simulink model "Final_integration_1"  (R2023b)
settings: Solver=FixedStepAuto  StartTime=0.0  StopTime=inf  FixedStep=Ts  RelTol=1e-3  EnableMultiTasking=on
InitFcn:
  | params
  | pin_params
undefined symbols (not defined in the file or in its folder): b, default1, den_Gd, encoder_scale, f, J, Kb, KD, Kf, KI, Km, KP, L, l, num_Gd, R, r, steering, Vlim
libraries: arduinolib x13, simulink x2, arduinosensorlib x2
settings Model: ExtModeTrigDuration=2  Creator=SJ  LastModifiedBy=SJ
settings SolverCC: AutoInsertRateTranBlk=on
settings OptimizationCC: EnhancedBackFolding=on  PassReuseOutputArgsAs=Individual arguments  ZeroExternalMemoryAtStartup=off  ZeroInternalMemoryAtStartup=off  MaxStackSize=64  OptimizeBlockOrder=speed  DifferentSizesBufferReuse=on  OptimizationCustomize=off  EfficientTunableParamExpr=on
settings DebuggingCC: ParameterTunabilityLossMsg=error
settings HardwareCC: ProdBitPerInt=16  ProdBitPerPointer=16  ProdBitPerSizeT=16  ProdBitPerPtrDiffT=16  ProdLargestAtomicFloat=None  ProdWordSize=8  ProdHWDeviceType=Atmel->AVR
settings SFSimCC: MATLABDynamicMemAlloc=off
settings RTWCC: Description=Embedded Coder  SystemTargetFile=ert.tlc  HardwareBoard=Arduino Mega 2560  TemplateMakefile=ert_default_tmf  Toolchain=Arduino AVR  BuildConfiguration=Faster Runs
settings CodeAppCC: ForceParamTrailComments=on  IgnoreCustomStorageClasses=off  OperatorAnnotations=on  SimulinkDataObjDesc=on  SFDataObjDesc=on  InsertBlockDesc=on
settings ERTTargetCC: SupportContinuousTime=on  SupportVariableSizeSignals=on  ExtModeTransport=3  ExtModeStaticAlloc=on  ExtModeAutomaticAllocSize=off  ExtModeStaticAllocSize=2048  ExtModeMexFile=ext_xcp  ExtModeIntrfLevel=Level2 - Open

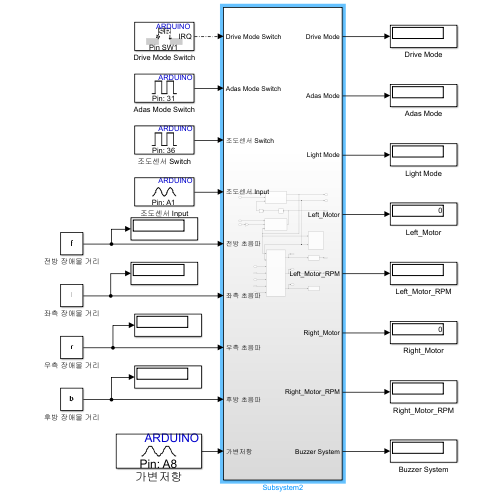
[thumbnail: Simulink's stored preview of the top-level diagram]
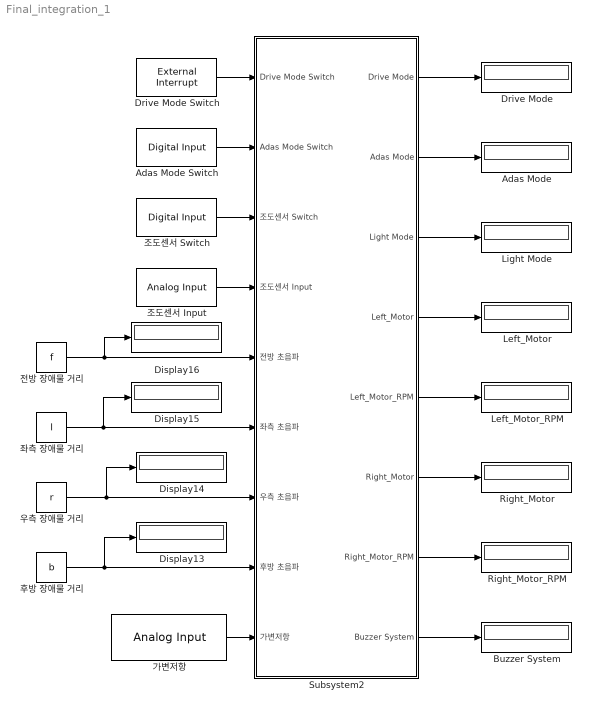
== system Final_integration_1 ==
  Adas Mode : Display
  Adas Mode Switch : arduinolib/Digital Input  pinNumber=SW2  mode=Default  Direction=input  SampleTime=0.01  blockPlatform=arduino
  Buzzer System : Display
  Display{13..16} (4 alike) : Display
  Drive Mode : Display
  Drive Mode Switch : arduinolib/External Interrupt  Pin=SW1  PullUp=off  Mode=RISING  InterruptSimulationInput=off
  Left_Motor : Display
  Left_Motor_RPM : Display
  Light Mode : Display
  Right_Motor : Display
  Right_Motor_RPM : Display
  Subsystem2 : Subsystem
  가변저항 : arduinolib/Analog Input  pinNumber=VR  ReadResultsOnly=off  ConversionTriggerSource=Software  ExternalTriggerType=uint32( 0 )  OutputDataType=uint16  EnableConversionCompleteNotify=off  EnableOuputStatus=off  SampleTime=-1  blockPlatform=arduino
  우측 장애물 거리 : Constant  Value=r
  전방 장애물 거리 : Constant  Value=f
  조도센서 Input : arduinolib/Analog Input  pinNumber=BS  ReadResultsOnly=off  ConversionTriggerSource=Software  ExternalTriggerType=uint32( 0 )  OutputDataType=uint16  EnableConversionCompleteNotify=off  EnableOuputStatus=off  SampleTime=0.01  blockPlatform=arduino
  조도센서 Switch : arduinolib/Digital Input  pinNumber=SW3  mode=Default  Direction=input  SampleTime=0.01  blockPlatform=arduino
  좌측 장애물 거리 : Constant  Value=l
  후방 장애물 거리 : Constant  Value=b
  wires:
  좌측 장애물 거리/1 -> Display15/1, Subsystem2/6(좌측 초음파)
  Subsystem2/7(Right_Motor_RPM) -> Right_Motor_RPM/1
  조도센서 Switch/1 -> Subsystem2/3(조도센서 Switch)
  우측 장애물 거리/1 -> Subsystem2/7(우측 초음파), Display14/1
  가변저항/1 -> Subsystem2/9(가변저항)
  전방 장애물 거리/1 -> Display16/1, Subsystem2/5(전방 초음파)
  조도센서 Input/1 -> Subsystem2/4(조도센서 Input)
  Subsystem2/3(Light Mode) -> Light Mode/1
  Subsystem2/8(Buzzer System) -> Buzzer System/1
  후방 장애물 거리/1 -> Display13/1, Subsystem2/8(후방 초음파)
  Adas Mode Switch/1 -> Subsystem2/2(Adas Mode Switch)
  Subsystem2/4(Left_Motor) -> Left_Motor/1
  Subsystem2/6(Right_Motor) -> Right_Motor/1
  Drive Mode Switch/1 -> Subsystem2/1(Drive Mode Switch)
  Subsystem2/5(Left_Motor_RPM) -> Left_Motor_RPM/1
  Subsystem2/2(Adas Mode) -> Adas Mode/1
  Subsystem2/1(Drive Mode) -> Drive Mode/1

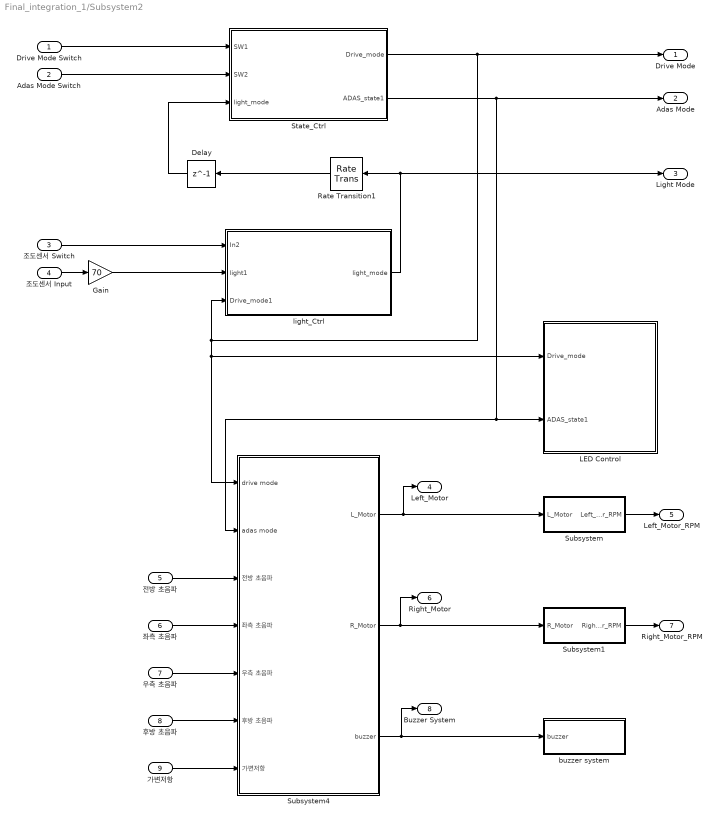
== system Final_integration_1/Subsystem2 ==
  Drive Mode Switch : Inport
  Adas Mode Switch : Inport  Port=2
  조도센서 Switch : Inport  Port=3
  조도센서 Input : Inport  Port=4
  전방 초음파 : Inport  Port=5
  좌측 초음파 : Inport  Port=6
  우측 초음파 : Inport  Port=7
  후방 초음파 : Inport  Port=8
  가변저항 : Inport  Port=9
  Delay : Delay  DelayLength=1
  Gain : Gain  Gain=70
  LED Control : Subsystem
  Rate Transition1 : RateTransition  Integrity=off
  State_Ctrl : Subsystem
  Subsystem : Subsystem
  Subsystem1 : Subsystem
  Subsystem4 : Subsystem
  buzzer system : Subsystem
  light_Ctrl : Subsystem
  Drive Mode : Outport
  Adas Mode : Outport  Port=2
  Light Mode : Outport  Port=3
  Left_Motor : Outport  Port=4
  Left_Motor_RPM : Outport  Port=5
  Right_Motor : Outport  Port=6
  Right_Motor_RPM : Outport  Port=7
  Buzzer System : Outport  Port=8
  wires:
  Subsystem4/1(L_Motor) -> Left_Motor/1, Subsystem/1(L_Motor)
  Subsystem4/3(buzzer) -> Buzzer System/1, buzzer system/1(buzzer)
  light_Ctrl/1(light_mode) -> Rate Transition1/1, Light Mode/1
  Gain/1 -> light_Ctrl/2(light1)
  Rate Transition1/1 -> Delay/1
  Drive Mode Switch/1 -> State_Ctrl/1(SW1)
  Delay/1 -> State_Ctrl/3(light_mode)
  Subsystem4/2(R_Motor) -> Right_Motor/1, Subsystem1/1(R_Motor)
  조도센서 Switch/1 -> light_Ctrl/1(In2)
  Adas Mode Switch/1 -> State_Ctrl/2(SW2)
  조도센서 Input/1 -> Gain/1
  전방 초음파/1 -> Subsystem4/3(전방 초음파)
  가변저항/1 -> Subsystem4/7(가변저항)
  후방 초음파/1 -> Subsystem4/6(후방 초음파)
  좌측 초음파/1 -> Subsystem4/4(좌측 초음파)
  우측 초음파/1 -> Subsystem4/5(우측 초음파)
  Subsystem/1(Left_Motor_RPM) -> Left_Motor_RPM/1
  Subsystem1/1(Right_Motor_RPM) -> Right_Motor_RPM/1
  State_Ctrl/1(Drive_mode) -> Drive Mode/1, Subsystem4/1(drive mode), LED Control/1(Drive_mode), light_Ctrl/3(Drive_mode1)
  State_Ctrl/2(ADAS_state1) -> Subsystem4/2(adas mode), LED Control/2(ADAS_state1), Adas Mode/1

== system Final_integration_1/Subsystem2/LED Control ==
  Drive_mode : Inport
  ADAS_state1 : Inport  Port=2
  LED_B Ctrl : Subsystem
  LED_R Ctrl : Subsystem
  wires:
  ADAS_state1/1 -> LED_B Ctrl/1(ADAS_state)
  Drive_mode/1 -> LED_B Ctrl/2(Drive_mode), LED_R Ctrl/1(Drive_mode)

== system Final_integration_1/Subsystem2/State_Ctrl ==
  SW1 : Inport
  SW2 : Inport  Port=2
  light_mode : Inport  Port=3
  ADAS_state : Subsystem
  Delay : Delay  DelayLength=1
  If : If  IfExpression=u1 ==1  ShowElse=off
  Rate Transition2 : RateTransition  Integrity=off  OutPortSampleTime=0.01
  drive_mode : Subsystem
  Drive_mode : Outport
  ADAS_state1 : Outport  Port=2
  wires:
  If/1 -> ADAS_state/1(In1)
  drive_mode/1(D_mode) -> If/1, Drive_mode/1
  ADAS_state/1(ADAS_state) -> Delay/1, ADAS_state1/1
  SW1/1 -> drive_mode/2(sw1)
  Delay/1 -> drive_mode/3(A_state)
  light_mode/1 -> drive_mode/1(light_mode)
  SW2/1 -> Rate Transition2/1
  Rate Transition2/1 -> ADAS_state/2(In2)

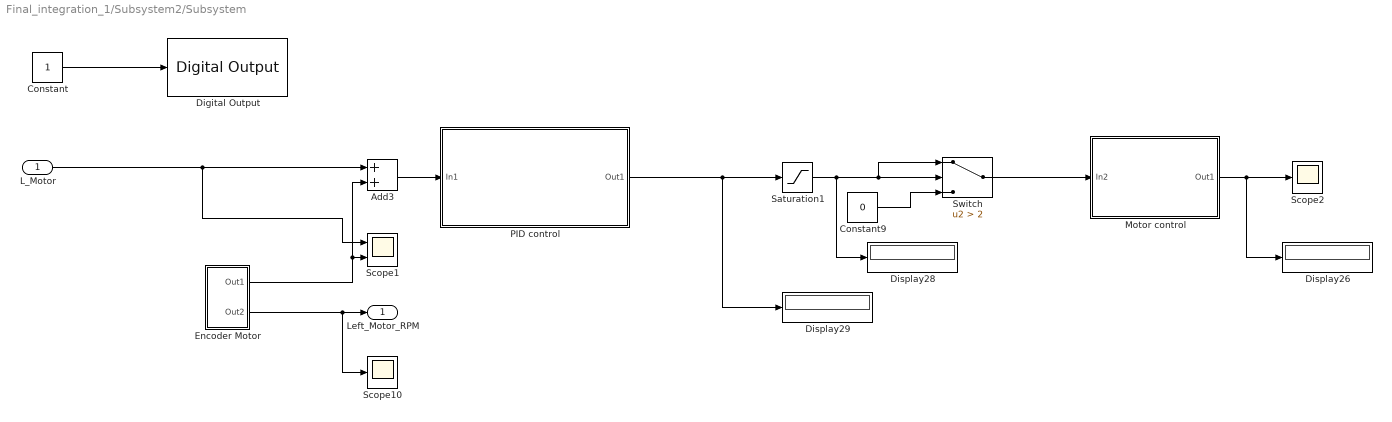
== system Final_integration_1/Subsystem2/Subsystem ==
  L_Motor : Inport
  Add3 : Sum
  Constant : Constant
  Constant9 : Constant  Value=0
  Digital Output : arduinolib/Digital Output  pinNumber=13  Direction=output  blockPlatform=arduino
  Display26 : Display
  Display28 : Display
  Display29 : Display
  Encoder Motor : Subsystem
  Motor control : Subsystem
  PID control : Subsystem
  Saturation1 : Saturate  UpperLimit=12  LowerLimit=2
  Scope1 : Scope  NumInputPorts=2
  Scope10 : Scope
  Scope2 : Scope
  Switch : Switch  Criteria=u2 > Threshold  Threshold=2  SaturateOnIntegerOverflow=off  InputSameDT=off
  Left_Motor_RPM : Outport
  wires:
  L_Motor/1 -> Scope1/1, Add3/1
  Encoder Motor/2(Out2) -> Left_Motor_RPM/1, Scope10/1
  Encoder Motor/1(Out1) -> Add3/2, Scope1/2
  Add3/1 -> PID control/1(In1)
  PID control/1(Out1) -> Display29/1, Saturation1/1
  Saturation1/1 -> Display28/1, Switch/1, Switch/2
  Switch/1 -> Motor control/1(In2)
  Constant9/1 -> Switch/3
  Motor control/1(Out1) -> Scope2/1, Display26/1
  Constant/1 -> Digital Output/1

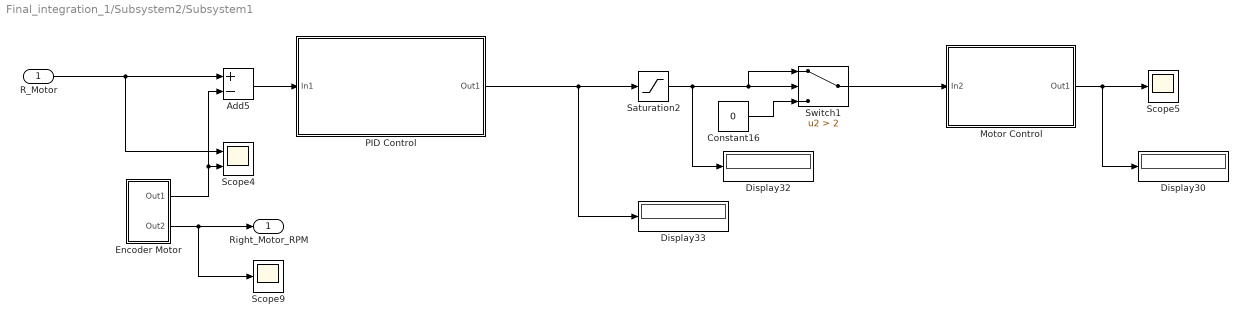
== system Final_integration_1/Subsystem2/Subsystem1 ==
  R_Motor : Inport
  Add5 : Sum  Inputs=+-
  Constant16 : Constant  Value=0
  Display30 : Display
  Display32 : Display
  Display33 : Display
  Encoder Motor : Subsystem
  Motor Control : Subsystem
  PID Control : Subsystem
  Saturation2 : Saturate  UpperLimit=12  LowerLimit=0
  Scope4 : Scope  NumInputPorts=2
  Scope5 : Scope
  Scope9 : Scope
  Switch1 : Switch  Criteria=u2 > Threshold  Threshold=2  SaturateOnIntegerOverflow=off  InputSameDT=off
  Right_Motor_RPM : Outport
  wires:
  Constant16/1 -> Switch1/3
  Switch1/1 -> Motor Control/1(In2)
  Saturation2/1 -> Switch1/1, Switch1/2, Display32/1
  Add5/1 -> PID Control/1(In1)
  R_Motor/1 -> Scope4/1, Add5/1
  Encoder Motor/1(Out1) -> Add5/2, Scope4/2
  PID Control/1(Out1) -> Display33/1, Saturation2/1
  Encoder Motor/2(Out2) -> Right_Motor_RPM/1, Scope9/1
  Motor Control/1(Out1) -> Scope5/1, Display30/1

== system Final_integration_1/Subsystem2/Subsystem4 ==
  drive mode : Inport
  adas mode : Inport  Port=2
  전방 초음파 : Inport  Port=3
  좌측 초음파 : Inport  Port=4
  우측 초음파 : Inport  Port=5
  후방 초음파 : Inport  Port=6
  가변저항 : Inport  Port=7
  Data Type Conversion : DataTypeConversion  OutDataTypeStr=double  SaturateOnIntegerOverflow=off  RndMeth=Floor
  Gain4 : Gain  Gain=0.25
  Subsystem : Subsystem
  L_Motor : Outport
  R_Motor : Outport  Port=2
  buzzer : Outport  Port=3
  wires:
  drive mode/1 -> Subsystem/1(DRIVE MODE1)
  adas mode/1 -> Subsystem/2(ADAS MODE1)
  Subsystem/3(buzzer) -> buzzer/1
  가변저항/1 -> Gain4/1
  Gain4/1 -> Data Type Conversion/1
  Data Type Conversion/1 -> Subsystem/7(가변저항1)
  Subsystem/2(R_Motor1) -> R_Motor/1
  Subsystem/1(L_Motor1) -> L_Motor/1
  전방 초음파/1 -> Subsystem/3(전방 초음파1)
  좌측 초음파/1 -> Subsystem/4(좌측 초음파1)
  우측 초음파/1 -> Subsystem/5(우측 초음파1)
  후방 초음파/1 -> Subsystem/6(후방 초음파1)

== system Final_integration_1/Subsystem2/buzzer system ==
  buzzer : Inport
  If : If  IfExpression=u1 == 1
  If Action Subsystem : Subsystem  TreatAsAtomicUnit=on
  If Action Subsystem1 : Subsystem  TreatAsAtomicUnit=on
  Merge : Merge
  PWM : arduinolib/PWM  pinNumber=Buzzer  frequencyType=Default  desiredFrequency=490.2  achievableFrequency=490.2
  wires:
  buzzer/1 -> If/1
  If/1 -> If Action Subsystem/Action
  If/2 -> If Action Subsystem1/Action
  If Action Subsystem/1(Output) -> Merge/1
  If Action Subsystem1/1(Out1) -> Merge/2
  Merge/1 -> PWM/1

== system Final_integration_1/Subsystem2/light_Ctrl ==
  In2 : Inport
  light1 : Inport  Port=2
  Drive_mode1 : Inport  Port=3
  If : If  IfExpression=u1 == 0  ShowElse=off
  If Action Subsystem : Subsystem  TreatAsAtomicUnit=on
  Rate Transition : RateTransition  Integrity=off
  Rate Transition1 : RateTransition  Integrity=off  OutPortSampleTime=0.2
  Subsystem : Subsystem
  light_mode : Outport
  wires:
  If Action Subsystem/1(light_mode) -> Rate Transition/1
  In2/1 -> Rate Transition1/1
  Rate Transition/1 -> Subsystem/2(light)
  Drive_mode1/1 -> If Action Subsystem/1(Drive_mode1)
  light1/1 -> Subsystem/1(light1)
  Subsystem/1(light_mode) -> light_mode/1
  If/1 -> If Action Subsystem/Action
  Rate Transition1/1 -> If/1

== system Final_integration_1/Subsystem2/LED Control/LED_B Ctrl ==
  ADAS_state : Inport
  Drive_mode : Inport  Port=2
  Constant : Constant
  Digital Output : arduinolib/Digital Output  pinNumber=LED1_B  Direction=output  blockPlatform=arduino
  If Action Subsystem1 : Subsystem  TreatAsAtomicUnit=on
  If Action Subsystem3 : Subsystem  TreatAsAtomicUnit=on
  If1 : If  IfExpression=u1 ==1
  Merge : Merge
  Product : Product
  Product1 : Product
  Pulse Generator : DiscretePulseGenerator  PulseType=Time based  PulseWidth=50
  wires:
  If1/2 -> If Action Subsystem3/Action
  If Action Subsystem1/1(Out1) -> Merge/1
  ADAS_state/1 -> If1/1
  If1/1 -> If Action Subsystem1/Action
  Merge/1 -> Digital Output/1
  If Action Subsystem3/1(Out1) -> Merge/2
  Drive_mode/1 -> Product/1, Product1/2
  Pulse Generator/1 -> Product/2
  Constant/1 -> Product1/1
  Product1/1 -> If Action Subsystem1/1(Input)
  Product/1 -> If Action Subsystem3/1(Input)

== system Final_integration_1/Subsystem2/LED Control/LED_R Ctrl ==
  Drive_mode : Inport
  Digital Output : arduinolib/Digital Output  pinNumber=LED1_R  Direction=output  blockPlatform=arduino
  If Action Subsystem1 : Subsystem  TreatAsAtomicUnit=on
  If Action Subsystem3 : Subsystem  TreatAsAtomicUnit=on
  If1 : If  IfExpression=u1 ==1
  Merge : Merge
  wires:
  If1/2 -> If Action Subsystem3/Action
  If Action Subsystem1/1(Out1) -> Merge/1
  Drive_mode/1 -> If1/1
  If1/1 -> If Action Subsystem1/Action
  Merge/1 -> Digital Output/1
  If Action Subsystem3/1(Out1) -> Merge/2

== system Final_integration_1/Subsystem2/State_Ctrl/ADAS_state ==
  In1 : Inport
  In2 : Inport  Port=2
  If : If  IfExpression=u1 == 0  ShowElse=off
  If Action Subsystem : Subsystem  TreatAsAtomicUnit=on
  If Action Subsystem1 : Subsystem  TreatAsAtomicUnit=on
  Rate Transition : RateTransition  Integrity=off
  Rate Transition2 : RateTransition  Integrity=off  OutPortSampleTime=0.2
  ADAS_state : Outport
  wires:
  In1/1 -> If Action Subsystem/Action
  If Action Subsystem/1(ADAS_state) -> ADAS_state/1
  In2/1 -> Rate Transition2/1
  Rate Transition2/1 -> If/1
  If/1 -> If Action Subsystem1/Action
  If Action Subsystem1/1(sw2) -> Rate Transition/1
  Rate Transition/1 -> If Action Subsystem/1(sw2)

== system Final_integration_1/Subsystem2/State_Ctrl/drive_mode ==
  light_mode : Inport
  sw1 : Inport  Port=2
  A_state : Inport  Port=3
  Rate Transition : RateTransition  Integrity=off  OutPortSampleTime=0.01
  Rate Transition1 : RateTransition  Integrity=off
  Rate Transition2 : RateTransition  Integrity=off
  SW1 : Subsystem
  D_mode : Outport
  wires:
  SW1/1(Output) -> Rate Transition/1
  sw1/1 -> SW1/Trigger
  Rate Transition/1 -> D_mode/1
  light_mode/1 -> Rate Transition1/1
  A_state/1 -> Rate Transition2/1
  Rate Transition1/1 -> SW1/1(light_mode)
  Rate Transition2/1 -> SW1/2(A_state)

== system Final_integration_1/Subsystem2/Subsystem/Encoder Motor ==
  Data Type Conversion1 : DataTypeConversion  OutDataTypeStr=int32  SaturateOnIntegerOverflow=off  RndMeth=Floor
  Discrete Transfer Fcn : DiscreteTransferFcn  Numerator=num_Gd  Denominator=den_Gd
  Discrete Derivative : simulink/Discrete/Discrete Derivative  gainval=1.0  ICPrevScaledInput=0.0  OutMin=[]  OutMax=[]  OutDataType=fixdt(1, 16)  OutScaling=2^-10  DoSatur=off
  Display : Display
  Encoder : arduinosensorlib/Encoder  InputA=L_Encoder_A  InputB=L_Encoder_B  Mode=No reset  SampleTime=0.01
  Gain1 : Gain  Gain=encoder_scale
  Gain2 : Gain  Gain=60/(2*pi)
  Out1 : Outport
  Out2 : Outport  Port=2
  wires:
  Gain1/1 -> Display/1, Gain2/1, Data Type Conversion1/1
  Encoder/1 -> Discrete Derivative/1
  Gain2/1 -> Out2/1
  Data Type Conversion1/1 -> Discrete Transfer Fcn/1
  Discrete Derivative/1 -> Gain1/1
  Discrete Transfer Fcn/1 -> Out1/1

== system Final_integration_1/Subsystem2/Subsystem/Motor control ==
  In2 : Inport
  Add : Sum  Commented=on  Inputs=+-
  Add1 : Sum  Commented=on
  Data Type Conversion : DataTypeConversion  OutDataTypeStr=uint8  SaturateOnIntegerOverflow=off  RndMeth=Floor
  Data Type Conversion1 : DataTypeConversion  OutDataTypeStr=double  SaturateOnIntegerOverflow=off  RndMeth=Floor
  Display1 : Display
  Gain : Gain  Commented=on  Gain=Kb
  Gain1 : Gain  Gain=255/Vlim
  PWM : arduinolib/PWM  pinNumber=Motor_L_Control  frequencyType=Default  desiredFrequency=490.2  achievableFrequency=490.2
  Transfer Fcn : TransferFcn  Commented=on  Numerator=Km  Denominator=[L R]
  Transfer Fcn1 : TransferFcn  Commented=on  Numerator=1  Denominator=[J Kf]
  Out1 : Outport
  wires:
  Add/1 -> Transfer Fcn/1
  Add1/1 -> Transfer Fcn1/1
  Transfer Fcn/1 -> Add1/2
  Gain/1 -> Add/2
  Transfer Fcn1/1 -> Gain/1
  In2/1 -> Gain1/1
  Gain1/1 -> Data Type Conversion/1
  Data Type Conversion1/1 -> Out1/1
  Data Type Conversion/1 -> Data Type Conversion1/1, Display1/1, PWM/1

== system Final_integration_1/Subsystem2/Subsystem/PID control ==
  In1 : Inport
  Add4 : Sum
  Derivative2 : Derivative  Commented=on
  Gain1 : Gain  Commented=on  Gain=KI
  Gain2 : Gain  Commented=on  Gain=KP
  Gain3 : Gain  Commented=on  Gain=KD
  Gain4 : Gain  Gain=KP
  Integrator2 : Integrator  Commented=on
  Subtract2 : Sum  Commented=on  Inputs=+++
  Transfer Fcn1 : TransferFcn  Numerator=[KI]  Denominator=[1 0]
  Out1 : Outport
  wires:
  Add4/1 -> Out1/1
  Gain4/1 -> Add4/2
  Transfer Fcn1/1 -> Add4/1
  Derivative2/1 -> Subtract2/3
  ? -> Gain2/1, Gain3/1, Gain1/1
  Integrator2/1 -> Subtract2/1
  Gain2/1 -> Subtract2/2
  Gain3/1 -> Derivative2/1
  Gain1/1 -> Integrator2/1
  In1/1 -> Gain4/1, Transfer Fcn1/1

== system Final_integration_1/Subsystem2/Subsystem1/Encoder Motor ==
  Data Type Conversion1 : DataTypeConversion  OutDataTypeStr=int32  SaturateOnIntegerOverflow=off  RndMeth=Floor
  Discrete Transfer Fcn : DiscreteTransferFcn  Numerator=num_Gd  Denominator=den_Gd
  Discrete Derivative : simulink/Discrete/Discrete Derivative  gainval=1.0  ICPrevScaledInput=0.0  OutMin=[]  OutMax=[]  OutDataType=fixdt(1, 16)  OutScaling=2^-10  DoSatur=off
  Display : Display
  Encoder : arduinosensorlib/Encoder  InputA=R_Encoder_A  InputB=R_Encoder_B  Mode=No reset  SampleTime=0.01
  Gain1 : Gain  Gain=encoder_scale
  Gain2 : Gain  Gain=60/(2*pi)
  Out1 : Outport
  Out2 : Outport  Port=2
  wires:
  Gain1/1 -> Display/1, Gain2/1, Data Type Conversion1/1
  Encoder/1 -> Discrete Derivative/1
  Gain2/1 -> Out2/1
  Data Type Conversion1/1 -> Discrete Transfer Fcn/1
  Discrete Derivative/1 -> Gain1/1
  Discrete Transfer Fcn/1 -> Out1/1

== system Final_integration_1/Subsystem2/Subsystem1/Motor Control ==
  In2 : Inport
  Add : Sum  Commented=on  Inputs=+-
  Add1 : Sum  Commented=on
  Data Type Conversion : DataTypeConversion  OutDataTypeStr=uint8  SaturateOnIntegerOverflow=off  RndMeth=Floor
  Data Type Conversion1 : DataTypeConversion  OutDataTypeStr=double  SaturateOnIntegerOverflow=off  RndMeth=Floor
  Display1 : Display
  Gain : Gain  Commented=on  Gain=Kb
  Gain1 : Gain  Gain=255/Vlim
  PWM : arduinolib/PWM  pinNumber=Motor_R_control  frequencyType=Default  desiredFrequency=490.2  achievableFrequency=490.2
  Transfer Fcn : TransferFcn  Commented=on  Numerator=Km  Denominator=[L R]
  Transfer Fcn1 : TransferFcn  Commented=on  Numerator=1  Denominator=[J Kf]
  Out1 : Outport
  wires:
  Add/1 -> Transfer Fcn/1
  Add1/1 -> Transfer Fcn1/1
  Transfer Fcn/1 -> Add1/2
  Gain/1 -> Add/2
  Transfer Fcn1/1 -> Gain/1
  In2/1 -> Gain1/1
  Gain1/1 -> Data Type Conversion/1
  Data Type Conversion1/1 -> Out1/1
  Data Type Conversion/1 -> Data Type Conversion1/1, Display1/1, PWM/1

== system Final_integration_1/Subsystem2/Subsystem1/PID Control ==
  In1 : Inport
  Add4 : Sum
  Derivative2 : Derivative  Commented=on
  Gain1 : Gain  Commented=on  Gain=KI
  Gain2 : Gain  Commented=on  Gain=KP
  Gain3 : Gain  Commented=on  Gain=KD
  Gain4 : Gain  Gain=KP
  Integrator2 : Integrator  Commented=on
  Subtract2 : Sum  Commented=on  Inputs=+++
  Transfer Fcn1 : TransferFcn  Numerator=[KI]  Denominator=[1 0]
  Out1 : Outport
  wires:
  Add4/1 -> Out1/1
  Derivative2/1 -> Subtract2/3
  Gain3/1 -> Derivative2/1
  ? -> Gain2/1, Gain3/1, Gain1/1
  Gain2/1 -> Subtract2/2
  Gain1/1 -> Integrator2/1
  Integrator2/1 -> Subtract2/1
  Transfer Fcn1/1 -> Add4/1
  Gain4/1 -> Add4/2
  In1/1 -> Transfer Fcn1/1, Gain4/1

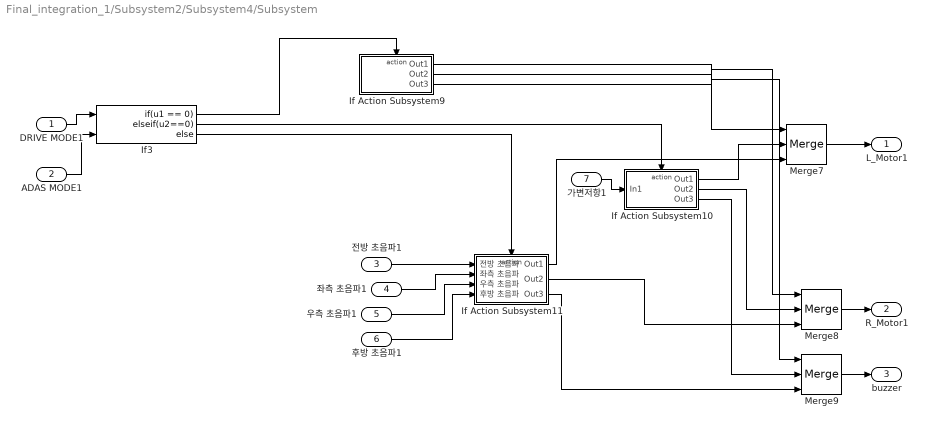
== system Final_integration_1/Subsystem2/Subsystem4/Subsystem ==
  DRIVE MODE1 : Inport
  ADAS MODE1 : Inport  Port=2
  전방 초음파1 : Inport  Port=3
  좌측 초음파1 : Inport  Port=4
  우측 초음파1 : Inport  Port=5
  후방 초음파1 : Inport  Port=6
  가변저항1 : Inport  Port=7
  If Action Subsystem10 : Subsystem  TreatAsAtomicUnit=on
  If Action Subsystem11 : Subsystem  TreatAsAtomicUnit=on
  If Action Subsystem9 : Subsystem  TreatAsAtomicUnit=on
  If3 : If  NumInputs=2  IfExpression=u1 == 0  ElseIfExpressions=u2==0
  Merge7 : Merge  Inputs=3
  Merge8 : Merge  Inputs=3
  Merge9 : Merge  Inputs=3
  L_Motor1 : Outport
  R_Motor1 : Outport  Port=2
  buzzer : Outport  Port=3
  wires:
  후방 초음파1/1 -> If Action Subsystem11/4(후방 초음파)
  Merge9/1 -> buzzer/1
  우측 초음파1/1 -> If Action Subsystem11/3(우측 초음파)
  If Action Subsystem11/1(Out1) -> Merge7/3
  Merge8/1 -> R_Motor1/1
  If Action Subsystem9/2(Out2) -> Merge8/1
  If3/3 -> If Action Subsystem11/Action
  If Action Subsystem10/1(Out1) -> Merge7/2
  Merge7/1 -> L_Motor1/1
  If3/1 -> If Action Subsystem9/Action
  If Action Subsystem9/1(Out1) -> Merge7/1
  If Action Subsystem9/3(Out3) -> Merge9/1
  좌측 초음파1/1 -> If Action Subsystem11/2(좌측 초음파)
  If Action Subsystem11/3(Out3) -> Merge9/3
  전방 초음파1/1 -> If Action Subsystem11/1(전방 초음파)
  If Action Subsystem10/2(Out2) -> Merge8/2
  If Action Subsystem10/3(Out3) -> Merge9/2
  If3/2 -> If Action Subsystem10/Action
  If Action Subsystem11/2(Out2) -> Merge8/3
  DRIVE MODE1/1 -> If3/1
  가변저항1/1 -> If Action Subsystem10/1(In1)
  ADAS MODE1/1 -> If3/2

== system Final_integration_1/Subsystem2/buzzer system/If Action Subsystem ==
  Action Port : ActionPort  ActionPortLabel=if(u1 == 1)
  Pulse Generator : DiscretePulseGenerator  PulseType=Time based  Period=0.2  PulseWidth=50
  Output : Outport
  wires:
  Pulse Generator/1 -> Output/1

== system Final_integration_1/Subsystem2/buzzer system/If Action Subsystem1 ==
  Action Port : ActionPort  ActionPortLabel=else
  Constant : Constant  Value=0
  Out1 : Outport
  wires:
  Constant/1 -> Out1/1

== system Final_integration_1/Subsystem2/light_Ctrl/If Action Subsystem ==
  Drive_mode1 : Inport
  Action Port : ActionPort  ActionPortLabel=if(u1 == 0)
  Constant : Constant
  Constant1 : Constant  Value=3
  Constant2 : Constant  Value=0
  Delay : Delay  DelayLength=1
  If : If  IfExpression=u1 == 1
  If Action Subsystem : Subsystem  TreatAsAtomicUnit=on
  If Action Subsystem1 : Subsystem  TreatAsAtomicUnit=on
  Merge : Merge
  Mod : Math  Operator=mod
  Plus : Sum
  light_mode : Outport
  wires:
  Mod/1 -> light_mode/1, Delay/1
  Delay/1 -> Plus/2
  Plus/1 -> Mod/1
  Constant1/1 -> Mod/2
  If/1 -> If Action Subsystem/Action
  If/2 -> If Action Subsystem1/Action
  Constant/1 -> If Action Subsystem/1(In1)
  Constant2/1 -> If Action Subsystem1/1(In1)
  If Action Subsystem/1(Out1) -> Merge/1
  If Action Subsystem1/1(Out1) -> Merge/2
  Merge/1 -> Plus/1
  Drive_mode1/1 -> If/1

== system Final_integration_1/Subsystem2/light_Ctrl/Subsystem ==
  light1 : Inport
  light : Inport  Port=2
  Chart1 : Stateflow chart  Commented=on  TreatAsAtomicUnit=on
  Subsystem : Subsystem
  light_mode : Outport
  wires:
  light1/1 -> Subsystem/1(light)
  light/1 -> light_mode/1, Subsystem/2(light_mode)

== system Final_integration_1/Subsystem2/LED Control/LED_B Ctrl/If Action Subsystem1 ==
  Input : Inport
  Action Port : ActionPort  ActionPortLabel=if(u1 ==1)
  Out1 : Outport
  wires:
  Input/1 -> Out1/1

== system Final_integration_1/Subsystem2/LED Control/LED_B Ctrl/If Action Subsystem3 ==
  Input : Inport
  Action Port : ActionPort  ActionPortLabel=else
  Out1 : Outport
  wires:
  Input/1 -> Out1/1

== system Final_integration_1/Subsystem2/LED Control/LED_R Ctrl/If Action Subsystem1 ==
  Action Port : ActionPort  ActionPortLabel=if(u1 ==1)
  Constant : Constant
  Out1 : Outport
  wires:
  Constant/1 -> Out1/1

== system Final_integration_1/Subsystem2/LED Control/LED_R Ctrl/If Action Subsystem3 ==
  Action Port : ActionPort  ActionPortLabel=else
  Constant : Constant  Value=0
  Out1 : Outport
  wires:
  Constant/1 -> Out1/1

== system Final_integration_1/Subsystem2/State_Ctrl/ADAS_state/If Action Subsystem ==
  sw2 : Inport
  Action Port : ActionPort  ActionPortLabel=if(u1 ==1)
  ADAS_state : Outport
  wires:
  sw2/1 -> ADAS_state/1

== system Final_integration_1/Subsystem2/State_Ctrl/ADAS_state/If Action Subsystem1 ==
  Action Port : ActionPort  ActionPortLabel=if(u1 == 0)
  Constant2 : Constant
  Constant3 : Constant  Value=2
  Delay1 : Delay  DelayLength=1  InitialCondition=0
  Mod1 : Math  Operator=mod
  Sum : Sum  Inputs=|++
  sw2 : Outport
  wires:
  Mod1/1 -> sw2/1
  Delay1/1 -> Sum/2
  Constant3/1 -> Mod1/2
  Sum/1 -> Delay1/1, Mod1/1
  Constant2/1 -> Sum/1

== system Final_integration_1/Subsystem2/State_Ctrl/drive_mode/SW1 ==
  light_mode : Inport
  A_state : Inport  Port=2
  function : TriggerPort  TriggerType=function-call  VariantControl=(inherit)
  Constant2 : Constant
  Delay : Delay  DelayLength=1
  If : If  IfExpression=u1 == 0  ElseIfExpressions=u1 == 1  ShowElse=off
  If Action Subsystem : Subsystem  TreatAsAtomicUnit=on
  If Action Subsystem1 : Subsystem  TreatAsAtomicUnit=on
  Merge : Merge
  Output : Outport
  wires:
  Delay/1 -> If/1
  If/1 -> If Action Subsystem/Action
  Constant2/1 -> If Action Subsystem/1(In1)
  If/2 -> If Action Subsystem1/Action
  If Action Subsystem/1(Out1) -> Merge/1
  light_mode/1 -> If Action Subsystem1/1(light_mode)
  A_state/1 -> If Action Subsystem1/2(A_state)
  If Action Subsystem1/1(Out1) -> Merge/2
  Merge/1 -> Delay/1, Output/1

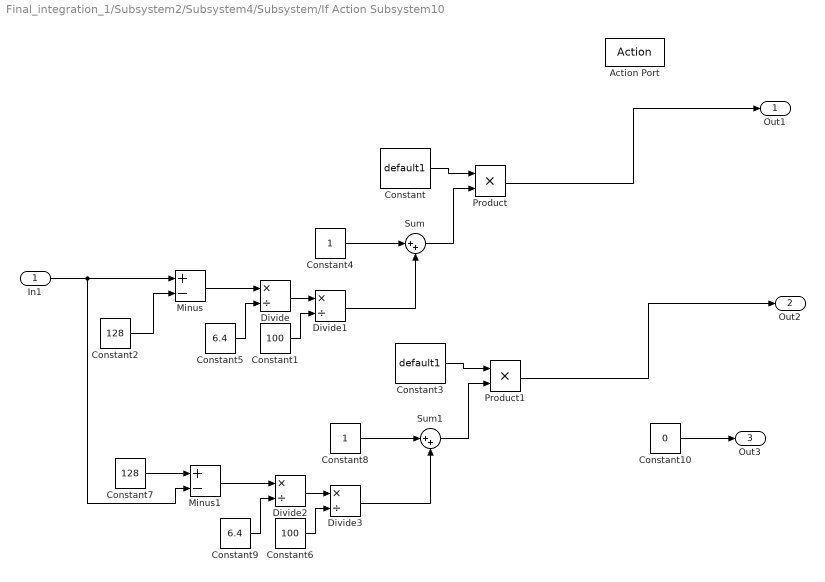
== system Final_integration_1/Subsystem2/Subsystem4/Subsystem/If Action Subsystem10 ==
  In1 : Inport
  Action Port : ActionPort  ActionPortLabel=elseif(u2==0)
  Constant : Constant  Value=default1
  Constant1 : Constant  Value=100
  Constant10 : Constant  Value=0
  Constant2 : Constant  Value=128
  Constant3 : Constant  Value=default1
  Constant4 : Constant
  Constant5 : Constant  Value=6.4
  Constant6 : Constant  Value=100
  Constant7 : Constant  Value=128
  Constant8 : Constant
  Constant9 : Constant  Value=6.4
  Divide{,1..3} (4 alike) : Product  Inputs=*/
  Minus : Sum  Inputs=+-
  Minus1 : Sum  Inputs=+-
  Product : Product
  Product1 : Product
  Sum : Sum  Inputs=|++
  Sum1 : Sum  Inputs=|++
  Out1 : Outport
  Out2 : Outport  Port=2
  Out3 : Outport  Port=3
  wires:
  Product/1 -> Out1/1
  Constant/1 -> Product/1
  In1/1 -> Minus/1, Minus1/2
  Constant2/1 -> Minus/2
  Minus/1 -> Divide/1
  Constant5/1 -> Divide/2
  Divide/1 -> Divide1/1
  Constant1/1 -> Divide1/2
  Constant4/1 -> Sum/1
  Divide1/1 -> Sum/2
  Sum/1 -> Product/2
  Constant7/1 -> Minus1/1
  Minus1/1 -> Divide2/1
  Constant3/1 -> Product1/1
  Constant9/1 -> Divide2/2
  Divide2/1 -> Divide3/1
  Divide3/1 -> Sum1/2
  Product1/1 -> Out2/1
  Constant6/1 -> Divide3/2
  Sum1/1 -> Product1/2
  Constant8/1 -> Sum1/1
  Constant10/1 -> Out3/1

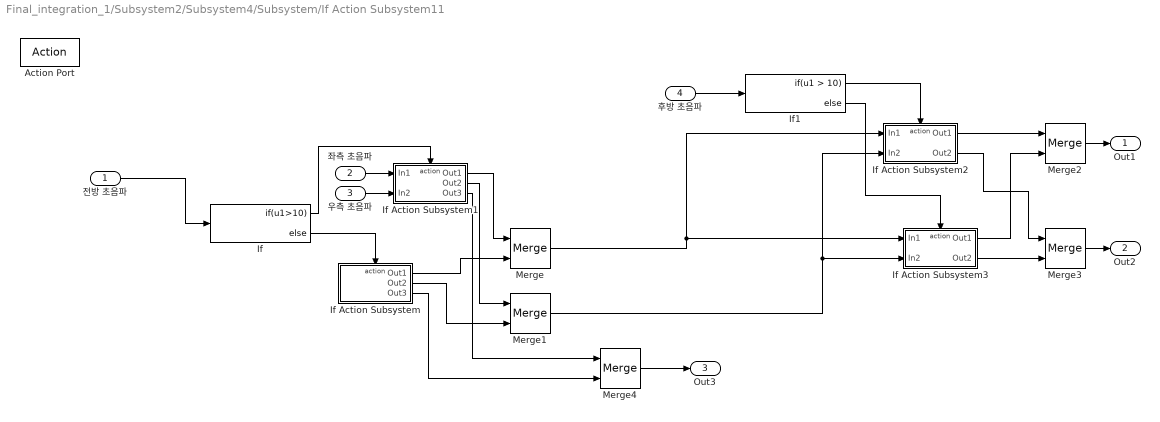
== system Final_integration_1/Subsystem2/Subsystem4/Subsystem/If Action Subsystem11 ==
  전방 초음파 : Inport
  좌측 초음파 : Inport  Port=2
  우측 초음파 : Inport  Port=3
  후방 초음파 : Inport  Port=4
  Action Port : ActionPort  ActionPortLabel=else
  If : If  IfExpression=u1>10
  If Action Subsystem : Subsystem  TreatAsAtomicUnit=on
  If Action Subsystem1 : Subsystem  TreatAsAtomicUnit=on
  If Action Subsystem2 : Subsystem  TreatAsAtomicUnit=on
  If Action Subsystem3 : Subsystem  TreatAsAtomicUnit=on
  If1 : If  IfExpression=u1 > 10
  Merge{,1..4} (5 alike) : Merge
  Out1 : Outport
  Out2 : Outport  Port=2
  Out3 : Outport  Port=3
  wires:
  If/2 -> If Action Subsystem/Action
  전방 초음파/1 -> If/1
  If/1 -> If Action Subsystem1/Action
  If Action Subsystem1/1(Out1) -> Merge/1
  If Action Subsystem/1(Out1) -> Merge/2
  Merge/1 -> If Action Subsystem3/1(In1), If Action Subsystem2/1(In1)
  If Action Subsystem1/2(Out2) -> Merge1/1
  If Action Subsystem/2(Out2) -> Merge1/2
  Merge1/1 -> If Action Subsystem3/2(In2), If Action Subsystem2/2(In2)
  좌측 초음파/1 -> If Action Subsystem1/1(In1)
  우측 초음파/1 -> If Action Subsystem1/2(In2)
  후방 초음파/1 -> If1/1
  If1/1 -> If Action Subsystem2/Action
  If1/2 -> If Action Subsystem3/Action
  If Action Subsystem2/1(Out1) -> Merge2/1
  If Action Subsystem3/1(Out1) -> Merge2/2
  If Action Subsystem3/2(Out2) -> Merge3/2
  If Action Subsystem2/2(Out2) -> Merge3/1
  Merge2/1 -> Out1/1
  Merge3/1 -> Out2/1
  If Action Subsystem1/3(Out3) -> Merge4/1
  If Action Subsystem/3(Out3) -> Merge4/2
  Merge4/1 -> Out3/1

== system Final_integration_1/Subsystem2/Subsystem4/Subsystem/If Action Subsystem9 ==
  Action Port : ActionPort  ActionPortLabel=if(u1 == 0)
  Constant : Constant  Value=0
  Out1 : Outport
  Out2 : Outport  Port=2
  Out3 : Outport  Port=3
  wires:
  Constant/1 -> Out3/1, Out2/1, Out1/1

== system Final_integration_1/Subsystem2/light_Ctrl/If Action Subsystem/If Action Subsystem ==
  In1 : Inport
  Action Port : ActionPort  ActionPortLabel=if(u1 == 1)
  Out1 : Outport
  wires:
  In1/1 -> Out1/1

== system Final_integration_1/Subsystem2/light_Ctrl/If Action Subsystem/If Action Subsystem1 ==
  In1 : Inport
  Action Port : ActionPort  ActionPortLabel=else
  Out1 : Outport
  wires:
  In1/1 -> Out1/1

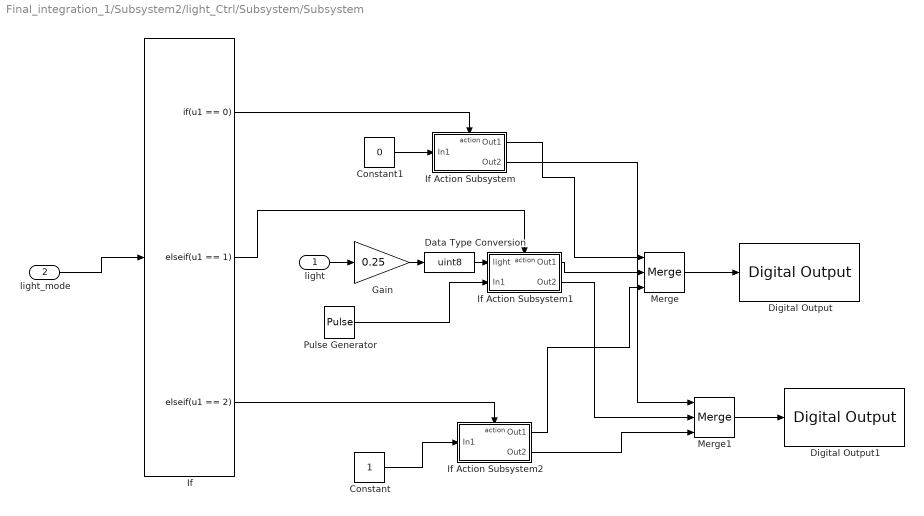
== system Final_integration_1/Subsystem2/light_Ctrl/Subsystem/Subsystem ==
  light : Inport
  light_mode : Inport  Port=2
  Constant : Constant
  Constant1 : Constant  Value=0
  Data Type Conversion : DataTypeConversion  OutDataTypeStr=uint8  SaturateOnIntegerOverflow=off  RndMeth=Floor
  Digital Output : arduinolib/Digital Output  pinNumber=LED2_R  Direction=output  blockPlatform=arduino
  Digital Output1 : arduinolib/Digital Output  pinNumber=LED2_B  Direction=output  blockPlatform=arduino
  Gain : Gain  Gain=0.25
  If : If  IfExpression=u1 == 0  ElseIfExpressions=u1 == 1, u1 == 2  ShowElse=off
  If Action Subsystem : Subsystem  TreatAsAtomicUnit=on
  If Action Subsystem1 : Subsystem  TreatAsAtomicUnit=on
  If Action Subsystem2 : Subsystem  TreatAsAtomicUnit=on
  Merge : Merge  Inputs=3
  Merge1 : Merge  Inputs=3
  Pulse Generator : DiscretePulseGenerator  PulseType=Time based  Period=0.2  PulseWidth=50
  wires:
  light_mode/1 -> If/1
  If/1 -> If Action Subsystem/Action
  If/2 -> If Action Subsystem1/Action
  If/3 -> If Action Subsystem2/Action
  Constant1/1 -> If Action Subsystem/1(In1)
  Constant/1 -> If Action Subsystem2/1(In1)
  If Action Subsystem/1(Out1) -> Merge/1
  If Action Subsystem1/1(Out1) -> Merge/2
  If Action Subsystem2/1(Out1) -> Merge/3
  Merge/1 -> Digital Output/1
  light/1 -> Gain/1
  Gain/1 -> Data Type Conversion/1
  Data Type Conversion/1 -> If Action Subsystem1/1(light)
  Pulse Generator/1 -> If Action Subsystem1/2(In1)
  If Action Subsystem1/2(Out2) -> Merge1/2
  If Action Subsystem/2(Out2) -> Merge1/1
  If Action Subsystem2/2(Out2) -> Merge1/3
  Merge1/1 -> Digital Output1/1

== system Final_integration_1/Subsystem2/State_Ctrl/drive_mode/SW1/If Action Subsystem ==
  In1 : Inport
  Action Port : ActionPort  ActionPortLabel=if(u1 == 0)
  Out1 : Outport
  wires:
  In1/1 -> Out1/1

== system Final_integration_1/Subsystem2/State_Ctrl/drive_mode/SW1/If Action Subsystem1 ==
  light_mode : Inport
  A_state : Inport  Port=2
  Action Port : ActionPort  ActionPortLabel=elseif(u1 == 1)
  Constant : Constant  Value=0
  Constant1 : Constant
  If Action Subsystem : Subsystem  TreatAsAtomicUnit=on
  If Action Subsystem1 : Subsystem  TreatAsAtomicUnit=on
  If1 : If  NumInputs=2  IfExpression=(u1 == 0) & (u2 == 0)
  Merge : Merge
  Out1 : Outport
  wires:
  A_state/1 -> If1/1
  light_mode/1 -> If1/2
  If1/1 -> If Action Subsystem1/Action
  Constant/1 -> If Action Subsystem1/1(In1)
  If1/2 -> If Action Subsystem/Action
  Constant1/1 -> If Action Subsystem/1(In1)
  If Action Subsystem1/1(Out1) -> Merge/1
  If Action Subsystem/1(Out1) -> Merge/2
  Merge/1 -> Out1/1

== system Final_integration_1/Subsystem2/Subsystem4/Subsystem/If Action Subsystem11/If Action Subsystem ==
  Action Port : ActionPort  ActionPortLabel=else
  Constant : Constant  Value=0
  Constant1 : Constant  Value=0
  Constant2 : Constant
  Out1 : Outport
  Out2 : Outport  Port=2
  Out3 : Outport  Port=3
  wires:
  Constant1/1 -> Out2/1
  Constant/1 -> Out1/1
  Constant2/1 -> Out3/1

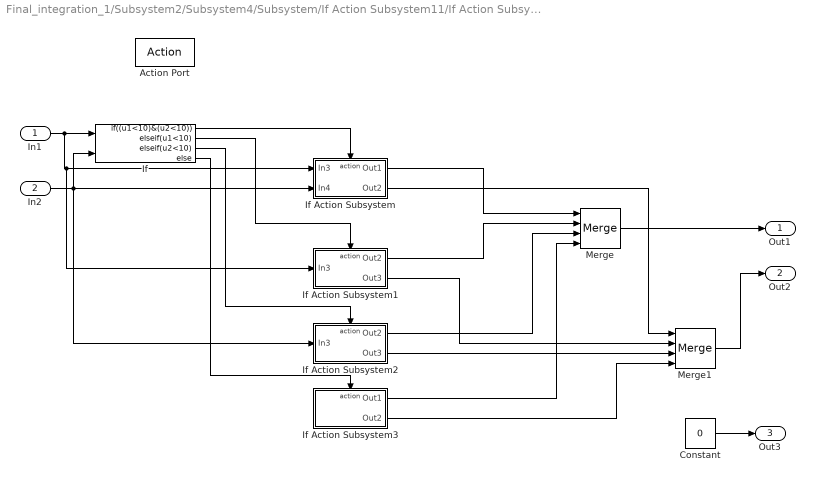
== system Final_integration_1/Subsystem2/Subsystem4/Subsystem/If Action Subsystem11/If Action Subsystem1 ==
  In1 : Inport
  In2 : Inport  Port=2
  Action Port : ActionPort  ActionPortLabel=if(u1>10)
  Constant : Constant  Value=0
  If : If  NumInputs=2  IfExpression=(u1<10)&(u2<10)  ElseIfExpressions=u1<10,u2<10
  If Action Subsystem : Subsystem  TreatAsAtomicUnit=on
  If Action Subsystem1 : Subsystem  TreatAsAtomicUnit=on
  If Action Subsystem2 : Subsystem  TreatAsAtomicUnit=on
  If Action Subsystem3 : Subsystem  TreatAsAtomicUnit=on
  Merge : Merge  Inputs=4
  Merge1 : Merge  Inputs=4
  Out1 : Outport
  Out2 : Outport  Port=2
  Out3 : Outport  Port=3
  wires:
  In1/1 -> If Action Subsystem1/1(In3), If Action Subsystem/1(In3), If/1
  If/1 -> If Action Subsystem/Action
  In2/1 -> If Action Subsystem2/1(In3), If Action Subsystem/2(In4), If/2
  If/2 -> If Action Subsystem1/Action
  If/3 -> If Action Subsystem2/Action
  If/4 -> If Action Subsystem3/Action
  If Action Subsystem/1(Out1) -> Merge/1
  If Action Subsystem1/1(Out2) -> Merge/2
  If Action Subsystem2/1(Out2) -> Merge/3
  If Action Subsystem3/1(Out1) -> Merge/4
  If Action Subsystem/2(Out2) -> Merge1/1
  If Action Subsystem1/2(Out3) -> Merge1/2
  If Action Subsystem2/2(Out3) -> Merge1/3
  If Action Subsystem3/2(Out2) -> Merge1/4
  Merge/1 -> Out1/1
  Merge1/1 -> Out2/1
  Constant/1 -> Out3/1

== system Final_integration_1/Subsystem2/Subsystem4/Subsystem/If Action Subsystem11/If Action Subsystem2 ==
  In1 : Inport
  In2 : Inport  Port=2
  Action Port : ActionPort  ActionPortLabel=if(u1 > 10)
  Out1 : Outport
  Out2 : Outport  Port=2
  wires:
  In1/1 -> Out1/1
  In2/1 -> Out2/1

== system Final_integration_1/Subsystem2/Subsystem4/Subsystem/If Action Subsystem11/If Action Subsystem3 ==
  In1 : Inport
  In2 : Inport  Port=2
  Action Port : ActionPort  ActionPortLabel=else
  Gain : Gain  Gain=1.2
  Gain1 : Gain  Gain=1.2
  Out1 : Outport
  Out2 : Outport  Port=2
  wires:
  In1/1 -> Gain/1
  Gain/1 -> Out1/1
  In2/1 -> Gain1/1
  Gain1/1 -> Out2/1

== system Final_integration_1/Subsystem2/light_Ctrl/Subsystem/Subsystem/If Action Subsystem ==
  In1 : Inport
  Action Port : ActionPort  ActionPortLabel=if(u1 == 0)
  Out1 : Outport
  Out2 : Outport  Port=2
  wires:
  In1/1 -> Out2/1, Out1/1

== system Final_integration_1/Subsystem2/light_Ctrl/Subsystem/Subsystem/If Action Subsystem1 ==
  light : Inport
  In1 : Inport  Port=2
  Action Port : ActionPort  ActionPortLabel=elseif(u1 == 1)
  Constant : Constant
  Constant1 : Constant  Value=0
  If : If  IfExpression=u1 <= 34
  If Action Subsystem : Subsystem  TreatAsAtomicUnit=on
  If Action Subsystem1 : Subsystem  TreatAsAtomicUnit=on
  Merge : Merge
  Out1 : Outport
  Out2 : Outport  Port=2
  wires:
  light/1 -> If/1
  Constant/1 -> If Action Subsystem/1(In1)
  Constant1/1 -> If Action Subsystem1/1(In1)
  If/1 -> If Action Subsystem/Action
  If/2 -> If Action Subsystem1/Action
  If Action Subsystem/1(Out1) -> Merge/1
  If Action Subsystem1/1(Out1) -> Merge/2
  Merge/1 -> Out1/1
  In1/1 -> Out2/1

== system Final_integration_1/Subsystem2/light_Ctrl/Subsystem/Subsystem/If Action Subsystem2 ==
  In1 : Inport
  Action Port : ActionPort  ActionPortLabel=elseif( u1 == 2)
  Out1 : Outport
  Out2 : Outport  Port=2
  wires:
  In1/1 -> Out2/1, Out1/1

== system Final_integration_1/Subsystem2/State_Ctrl/drive_mode/SW1/If Action Subsystem1/If Action Subsystem ==
  In1 : Inport
  Action Port : ActionPort  ActionPortLabel=else
  Out1 : Outport
  wires:
  In1/1 -> Out1/1

== system Final_integration_1/Subsystem2/State_Ctrl/drive_mode/SW1/If Action Subsystem1/If Action Subsystem1 ==
  In1 : Inport
  Action Port : ActionPort  ActionPortLabel=if((u1 == 0) & (u2 == 0) )
  Out1 : Outport
  wires:
  In1/1 -> Out1/1

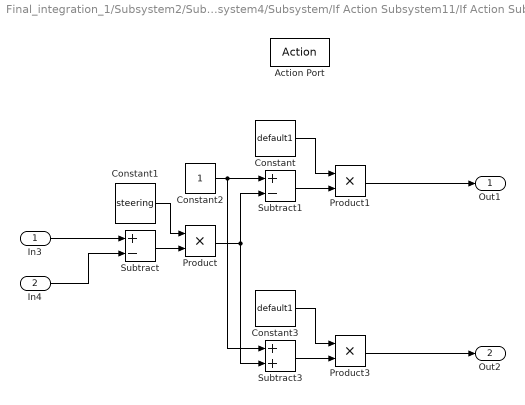
== system Final_integration_1/Subsystem2/Subsystem4/Subsystem/If Action Subsystem11/If Action Subsystem1/If Action Subsystem ==
  In3 : Inport
  In4 : Inport  Port=2
  Action Port : ActionPort  ActionPortLabel=if((u1<10)&(u2<10))
  Constant : Constant  Value=default1
  Constant1 : Constant  Value=steering
  Constant2 : Constant
  Constant3 : Constant  Value=default1
  Product : Product
  Product1 : Product
  Product3 : Product
  Subtract : Sum  Inputs=+-
  Subtract1 : Sum  Inputs=+-
  Subtract3 : Sum
  Out1 : Outport
  Out2 : Outport  Port=2
  wires:
  Subtract/1 -> Product/2
  Constant1/1 -> Product/1
  Subtract1/1 -> Product1/2
  Product/1 -> Subtract1/2, Subtract3/2
  Constant/1 -> Product1/1
  Product1/1 -> Out1/1
  Subtract3/1 -> Product3/2
  Constant2/1 -> Subtract3/1, Subtract1/1
  In4/1 -> Subtract/2
  Constant3/1 -> Product3/1
  In3/1 -> Subtract/1
  Product3/1 -> Out2/1

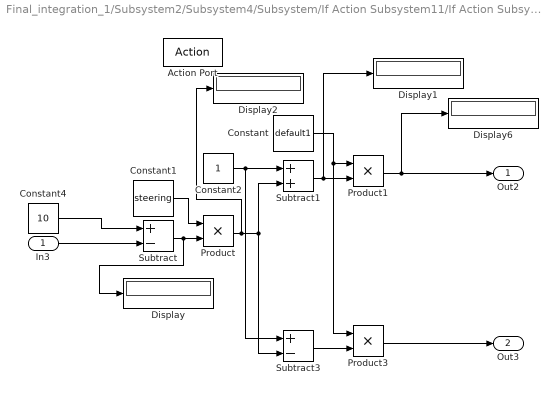
== system Final_integration_1/Subsystem2/Subsystem4/Subsystem/If Action Subsystem11/If Action Subsystem1/If Action Subsystem1 ==
  In3 : Inport
  Action Port : ActionPort  ActionPortLabel=elseif(u1<10)
  Constant : Constant  Value=default1
  Constant1 : Constant  Value=steering
  Constant2 : Constant
  Constant4 : Constant  Value=10
  Display{,1..2,6} (4 alike) : Display
  Product : Product  OutDataTypeStr=double  RndMeth=Convergent
  Product1 : Product  OutDataTypeStr=double  RndMeth=Convergent
  Product3 : Product  OutDataTypeStr=double  RndMeth=Convergent
  Subtract : Sum  Inputs=+-  OutDataTypeStr=double  RndMeth=Convergent
  Subtract1 : Sum  OutDataTypeStr=double  RndMeth=Convergent
  Subtract3 : Sum  Inputs=+-  OutDataTypeStr=double  RndMeth=Convergent
  Out2 : Outport
  Out3 : Outport  Port=2
  wires:
  Product/1 -> Display2/1, Subtract1/2, Subtract3/2
  Subtract1/1 -> Display1/1, Product1/2
  Constant1/1 -> Product/1
  Constant2/1 -> Subtract3/1, Subtract1/1
  In3/1 -> Subtract/2
  Subtract/1 -> Display/1, Product/2
  Subtract3/1 -> Product3/2
  Product3/1 -> Out3/1
  Constant/1 -> Product3/1, Product1/1
  Product1/1 -> Display6/1, Out2/1
  Constant4/1 -> Subtract/1

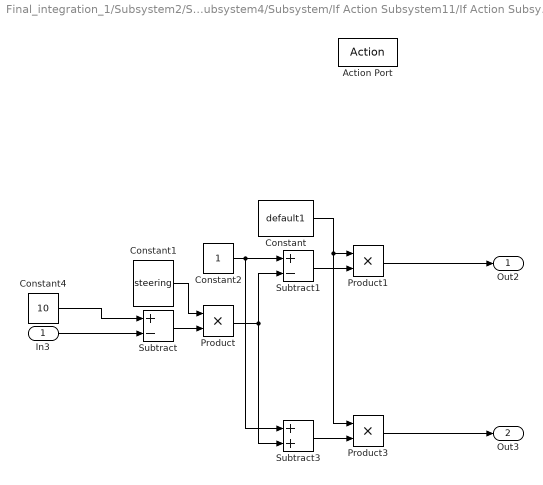
== system Final_integration_1/Subsystem2/Subsystem4/Subsystem/If Action Subsystem11/If Action Subsystem1/If Action Subsystem2 ==
  In3 : Inport
  Action Port : ActionPort  ActionPortLabel=elseif(u2<10)
  Constant : Constant  Value=default1
  Constant1 : Constant  Value=steering
  Constant2 : Constant
  Constant4 : Constant  Value=10
  Product : Product
  Product1 : Product
  Product3 : Product
  Subtract : Sum  Inputs=+-
  Subtract1 : Sum  Inputs=+-
  Subtract3 : Sum
  Out2 : Outport
  Out3 : Outport  Port=2
  wires:
  Constant4/1 -> Subtract/1
  Constant/1 -> Product3/1, Product1/1
  Product/1 -> Subtract1/2, Subtract3/2
  Product3/1 -> Out3/1
  Subtract3/1 -> Product3/2
  Subtract/1 -> Product/2
  Subtract1/1 -> Product1/2
  Product1/1 -> Out2/1
  Constant1/1 -> Product/1
  Constant2/1 -> Subtract3/1, Subtract1/1
  In3/1 -> Subtract/2

== system Final_integration_1/Subsystem2/Subsystem4/Subsystem/If Action Subsystem11/If Action Subsystem1/If Action Subsystem3 ==
  Action Port : ActionPort  ActionPortLabel=else
  Constant : Constant  Value=default1
  Constant1 : Constant  Value=default1
  Out1 : Outport
  Out2 : Outport  Port=2
  wires:
  Constant/1 -> Out1/1
  Constant1/1 -> Out2/1

== system Final_integration_1/Subsystem2/light_Ctrl/Subsystem/Subsystem/If Action Subsystem1/If Action Subsystem ==
  In1 : Inport
  Action Port : ActionPort  ActionPortLabel=if(u1 <= 34)
  Out1 : Outport
  wires:
  In1/1 -> Out1/1

== system Final_integration_1/Subsystem2/light_Ctrl/Subsystem/Subsystem/If Action Subsystem1/If Action Subsystem1 ==
  In1 : Inport
  Action Port : ActionPort  ActionPortLabel=else
  Out1 : Outport
  wires:
  In1/1 -> Out1/1

== stateflow chart Final_integration_1/Subsystem2/light_Ctrl/Subsystem/Chart1 ==
  state light_auto
    en, du:
    light_mode = 1;
    state_1 = sw3;
  state light_off
    en, du:
    light_mode =0;
    state_1 = sw3;
  state light_on
    en,du:
    light_mode =2;
    state_1 = sw3;
  light_auto -> (junction 15) : [(state_1 ~= sw3) && (Drive_mode == 1)]
  (junction 12) -> light_auto
  (junction 15) -> light_on
  light_off -> (junction 12) : [(state_1 ~= sw3) && (Drive_mode == 1)]
  (default) -> light_off
  light_on -> light_off : [(state_1 ~= sw3) && (Drive_mode == 1)]
  data: sw3 input; Drive_mode input; state_1 local; light_mode output
